simulink model "Multi_Scenario_WECS_based_Microgrid_2017"  (R2023a)
settings: Solver=ode45  StartTime=0.0  StopTime=4  RelTol=1e-3  EnableMultiTasking=on
undefined symbols (not defined in the file): c1, c2, c3, c4, c5, c6, DiscIntNeverNeededParam, fdesignblkfcn, gcbh, Hydride, Metal, Nickel
libraries: powerlib x63, powerlib_extras x26, powerlib_meascontrol x25, simulink x5, simulink_extras x2, electricdrivelib x1
(part 3 of 3)

== system Multi_Scenario_WECS_based_Microgrid_2017/Grid side control/Discrete PI Controller2 ==
  note: Discrete PID Controller
  note: Pierre Giroux, Gilbert Sybille
      | Power System Simulation Laboratory
      | IREQ, Hydro-Quebc
  Error : Inport  SampleTime=Ts
  Discrete-Time Integrator : DiscreteIntegrator  InitialCondition=Init  SampleTime=Ts  LimitOutput=on  UpperSaturationLimit=UpperLimit  LowerSaturationLimit=LowerLimit  ICPrevOutput=DiscIntNeverNeededParam  ICPrevScaledInput=DiscIntNeverNeededParam
  Kp4 : Gain  Gain=Kp  SaturateOnIntegerOverflow=on  SampleTime=Ts  OutDataTypeStr=Inherit: Same as input  ParamDataTypeStr=Inherit: Same as input
  Kp5 : Gain  Gain=Ki  SaturateOnIntegerOverflow=on  SampleTime=Ts  OutDataTypeStr=Inherit: Same as input  ParamDataTypeStr=Inherit: Same as input
  Saturation2 : Saturate  UpperLimit=UpperLimit  LowerLimit=LowerLimit  SampleTime=Ts
  Sum6 : Sum  InputSameDT=on  SaturateOnIntegerOverflow=on  SampleTime=Ts  OutDataTypeStr=Inherit: Same as first input
  Zero-Order Hold : ZeroOrderHold  SampleTime=Ts
  Out : Outport  SampleTime=Ts  InitialOutput=0
  wires:
  Zero-Order Hold/1 -> Sum6/1
  Saturation2/1 -> Out/1
  Discrete-Time Integrator/1 -> Sum6/2
  Kp4/1 -> Zero-Order Hold/1
  Kp5/1 -> Discrete-Time Integrator/1
  Sum6/1 -> Saturation2/1
  Error/1 -> Kp5/1, Kp4/1

== system Multi_Scenario_WECS_based_Microgrid_2017/Grid side control/Discrete PI Controller3 ==
  note: Pierre Giroux, Gilbert Sybille
      | Power System Simulation Laboratory
      | IREQ, Hydro-Quebc
  note: Discrete PID Controller
  Error : Inport  SampleTime=Ts
  Discrete-Time Integrator : DiscreteIntegrator  InitialCondition=Init  SampleTime=Ts  LimitOutput=on  UpperSaturationLimit=UpperLimit  LowerSaturationLimit=LowerLimit  ICPrevOutput=DiscIntNeverNeededParam  ICPrevScaledInput=DiscIntNeverNeededParam
  Kp4 : Gain  Gain=Kp  SaturateOnIntegerOverflow=on  SampleTime=Ts  OutDataTypeStr=Inherit: Same as input  ParamDataTypeStr=Inherit: Same as input
  Kp5 : Gain  Gain=Ki  SaturateOnIntegerOverflow=on  SampleTime=Ts  OutDataTypeStr=Inherit: Same as input  ParamDataTypeStr=Inherit: Same as input
  Saturation2 : Saturate  UpperLimit=UpperLimit  LowerLimit=LowerLimit  SampleTime=Ts
  Sum6 : Sum  InputSameDT=on  SaturateOnIntegerOverflow=on  SampleTime=Ts  OutDataTypeStr=Inherit: Same as first input
  Zero-Order Hold : ZeroOrderHold  SampleTime=Ts
  Out : Outport  SampleTime=Ts  InitialOutput=0
  wires:
  Error/1 -> Kp4/1, Kp5/1
  Sum6/1 -> Saturation2/1
  Kp5/1 -> Discrete-Time Integrator/1
  Kp4/1 -> Zero-Order Hold/1
  Discrete-Time Integrator/1 -> Sum6/2
  Saturation2/1 -> Out/1
  Zero-Order Hold/1 -> Sum6/1

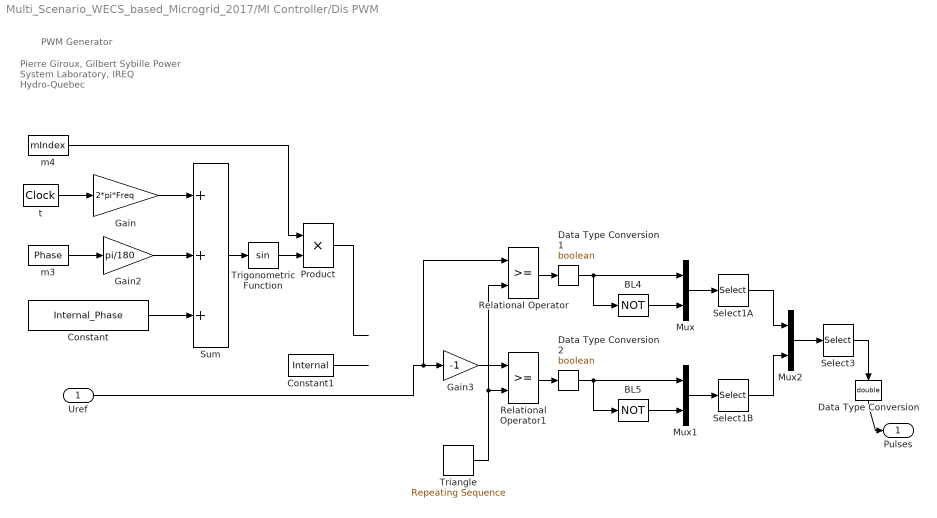
== system Multi_Scenario_WECS_based_Microgrid_2017/MI Controller/Dis PWM ==
  note: Pierre Giroux, Gilbert Sybille
      | Power System Laboratory, IREQ
      | Hydro-Quebec
  note: PWM Generator
  Uref : Inport
  BL4 : Logic  Operator=NOT  Inputs=1
  BL5 : Logic  Operator=NOT  Inputs=1
  Constant : Constant  Value=Internal_Phase
  Constant1 : Constant  Value=Internal
  Data Type Conversion : DataTypeConversion  OutDataTypeStr=double
  Data Type Conversion1 : DataTypeConversion  OutDataTypeStr=boolean
  Data Type Conversion2 : DataTypeConversion  OutDataTypeStr=boolean
  Gain : Gain  Gain=2*pi*Freq  SaturateOnIntegerOverflow=on  OutDataTypeStr=Inherit: Same as input  ParamDataTypeStr=Inherit: Same as input
  Gain2 : Gain  Gain=pi/180  SaturateOnIntegerOverflow=on  OutDataTypeStr=Inherit: Same as input  ParamDataTypeStr=Inherit: Same as input
  Gain3 : Gain  Gain=-1  SaturateOnIntegerOverflow=on  OutDataTypeStr=Inherit: Same as input  ParamDataTypeStr=Inherit: Same as input
  Mux : Mux  Inputs=2
  Mux1 : Mux  Inputs=2
  Mux2 : Mux  Inputs=2
  Product : Product  InputSameDT=on  SaturateOnIntegerOverflow=on  OutDataTypeStr=Inherit: Same as first input
  Relational Operator : RelationalOperator
  Relational Operator1 : RelationalOperator
  Select1A : Selector  InputPortWidth=Select1_PortWidth  IndexOptions=Index vector (dialog)  Indices=Select1_Elements  OutputSizes=1
  Select1B : Selector  InputPortWidth=Select1_PortWidth  IndexOptions=Index vector (dialog)  Indices=Select1_Elements  OutputSizes=1
  Select3 : Selector  InputPortWidth=Select3_PortWidth  IndexOptions=Index vector (dialog)  Indices=Select3_Elements  OutputSizes=1
  Sum : Sum  Inputs=+++  InputSameDT=on  SaturateOnIntegerOverflow=on  OutDataTypeStr=Inherit: Same as first input
  Triangle : simulink/Sources/Repeating Sequence  rep_seq_t=[0 1/Fc/4 3/Fc/4 1/Fc]  rep_seq_y=[0 -1 1 0]
  Trigonometric Function : Trigonometry
  m3 : Constant  Value=Phase
  m4 : Constant  Value=mIndex
  t : DigitalClock  SampleTime=Ts
  Pulses : Outport
  wires:
  Mux2/1 -> Select3/1
  Select1B/1 -> Mux2/2
  Select1A/1 -> Mux2/1
  Mux1/1 -> Select1B/1
  Mux/1 -> Select1A/1
  BL5/1 -> Mux1/2
  BL4/1 -> Mux/2
  Gain3/1 -> Relational Operator1/1
  Triangle/1 -> Relational Operator1/2, Relational Operator/2
  Product/1 -> ?
  Constant1/1 -> ?
  Uref/1 -> Relational Operator/1, Gain3/1
  Trigonometric Function/1 -> Product/2
  Sum/1 -> Trigonometric Function/1
  m4/1 -> Product/1
  Constant/1 -> Sum/3
  m3/1 -> Gain2/1
  Gain2/1 -> Sum/2
  Gain/1 -> Sum/1
  t/1 -> Gain/1
  Select3/1 -> Data Type Conversion/1
  Data Type Conversion/1 -> Pulses/1
  Relational Operator/1 -> Data Type Conversion1/1
  Data Type Conversion1/1 -> BL4/1, Mux/1
  Relational Operator1/1 -> Data Type Conversion2/1
  Data Type Conversion2/1 -> BL5/1, Mux1/1

== system Multi_Scenario_WECS_based_Microgrid_2017/MI Controller/Switch2 ==
  Vdq : Inport
  Compare To Constant1 : simulink/Logic and Bit Operations/Compare To Constant  relop=<  const=388  OutDataTypeStr=boolean
  Fcn1 : Fcn  Expr=sqrt(u(1)^2+u(2)^2)
  SW : Outport
  wires:
  Vdq/1 -> Fcn1/1
  Fcn1/1 -> Compare To Constant1/1
  Compare To Constant1/1 -> SW/1

== system Multi_Scenario_WECS_based_Microgrid_2017/MI Controller/central control ==
  Vdq_load : Inport
  Vdq_droop : Inport  Port=2
  Add1 : Sum
  Add2 : Sum
  Demux1 : Demux  Outputs=2
  Demux2 : Demux  Outputs=2
  Discrete PI Controller1 : powerlib_extras/Discrete  Control Blocks/Discrete PI Controller  Kp=0.2  Ki=40  Par_Limits=[100 -100]  Init=0  Ts=2e-05
  Discrete PI Controller2 : powerlib_extras/Discrete  Control Blocks/Discrete PI Controller  Kp=0.2  Ki=40  Par_Limits=[100 -100]  Init=0  Ts=2e-05
  Mux4 : Mux  Inputs=2
  Sum1 : Sum  Inputs=-+
  Sum2 : Sum  Inputs=-+
  v1 : Scope  NumInputPorts=2
  v5 : Scope  NumInputPorts=2
  out : Outport
  wires:
  Mux4/1 -> out/1
  Vdq_load/1 -> v1/1, Demux2/1
  Vdq_droop/1 -> v1/2, Demux1/1
  Demux2/1 -> Sum1/1
  Demux2/2 -> Sum2/1
  Sum1/1 -> Discrete PI Controller2/1
  Sum2/1 -> Discrete PI Controller1/1
  Demux1/2 -> Add2/2, Sum2/2
  Discrete PI Controller1/1 -> v5/2, Add2/1
  Discrete PI Controller2/1 -> v5/1, Add1/1
  Demux1/1 -> Add1/2, Sum1/2
  Add1/1 -> Mux4/1
  Add2/1 -> Mux4/2

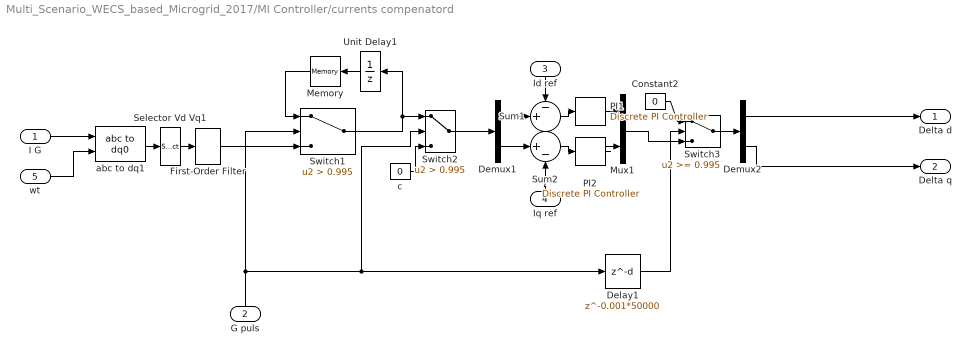
== system Multi_Scenario_WECS_based_Microgrid_2017/MI Controller/currents compenatord ==
  I G : Inport
  G puls : Inport  Port=2
  Id ref : Inport  Port=3
  Iq ref : Inport  Port=4
  wt : Inport  Port=5
  Constant2 : Constant  Value=0
  Delay1 : Delay  DelayLength=0.001*50000  InitialCondition=0  SampleTime=2e-05
  Demux1 : Demux  Outputs=2
  Demux2 : Demux  Outputs=2
  First-Order Filter : powerlib_meascontrol/Filters/First-Order Filter  FilterType=Lowpass  Tc=1e-3  Ts=0  Initialize=on  Vac_Init=[0, 0, 50]  Vdc_Init=0  PlotResponse=off  FreqRange="[0,  200,  1]"
  Memory : Memory
  Mux1 : Mux  Inputs=2
  "PI1 " : powerlib_extras/Discrete  Control Blocks/Discrete PI Controller  Kp=0.1  Ki=4  Par_Limits=[200 -200]  Init=0  Ts=2e-05
  PI2 : powerlib_extras/Discrete  Control Blocks/Discrete PI Controller  Kp=0.1  Ki=4  Par_Limits=[200 -200]  Init=0  Ts=2e-05
  Selector Vd Vq1 : Selector  InputPortWidth=3  IndexOptions=Index vector (dialog)  Indices=[1 2]  OutputSizes=1
  Sum1 : Sum  Inputs=-+|
  Sum2 : Sum  Inputs=|+-
  Switch1 : Switch  Criteria=u2 > Threshold  Threshold=0.995  SaturateOnIntegerOverflow=off  InputSameDT=off
  Switch2 : Switch  Criteria=u2 > Threshold  Threshold=0.995  SaturateOnIntegerOverflow=off  InputSameDT=off
  Switch3 : Switch  Threshold=0.995  SaturateOnIntegerOverflow=off  InputSameDT=off
  Unit Delay1 : UnitDelay  SampleTime=2e-05  HasFrameUpgradeWarning=on
  abc to dq1 : powerlib_meascontrol/Transformations/abc to dq0  Alignment=90 degrees behind phase A axis
  c : Constant  Value=0
  Delta d : Outport
  Delta q : Outport  Port=2
  wires:
  wt/1 -> abc to dq1/2
  Iq ref/1 -> Sum2/2
  Id ref/1 -> Sum1/1
  I G/1 -> abc to dq1/1
  abc to dq1/1 -> Selector Vd Vq1/1
  First-Order Filter/1 -> Switch1/3
  Switch1/1 -> Switch2/1, Unit Delay1/1
  Memory/1 -> Switch1/1
  Unit Delay1/1 -> Memory/1
  Demux1/1 -> Sum1/2
  Demux1/2 -> Sum2/1
  Sum2/1 -> PI2/1
  Sum1/1 -> "PI1 "/1
  Mux1/1 -> Switch3/3
  Demux2/1 -> Delta d/1
  Demux2/2 -> Delta q/1
  Switch3/1 -> Demux2/1
  Constant2/1 -> Switch3/1
  G puls/1 -> Switch2/2, Delay1/1, Switch1/2
  Selector Vd Vq1/1 -> First-Order Filter/1
  Delay1/1 -> Switch3/2
  "PI1 "/1 -> Mux1/1
  PI2/1 -> Mux1/2
  Switch2/1 -> Demux1/1
  c/1 -> Switch2/3

== system Multi_Scenario_WECS_based_Microgrid_2017/MI Controller/droop ==
  PQ : Inport
  Demux1 : Demux  Outputs=2
  Gain : Gain  Gain=2*pi
  Integrator : Integrator
  Pref : Constant  Value=180e3
  Subsystem1 : Subsystem
  Sum1 : Sum  Inputs=|+-
  Sum2 : Sum  Inputs=+-|
  Sum3 : Sum  Inputs=|-+
  Un : Constant  Value=390
  fn : Constant  Value=50
  m : Gain  Gain=6e-5
  n : Gain  Gain=4e-4
  Vabc : Outport
  wt : Outport  Port=2
  wires:
  Sum1/1 -> m/1
  fn/1 -> Sum2/1
  n/1 -> Sum2/2
  Sum2/1 -> Gain/1  "f"
  m/1 -> Sum3/1
  Un/1 -> Sum3/2
  Sum3/1 -> Subsystem1/2(Uref)
  Gain/1 -> Integrator/1  "w"
  Pref/1 -> Sum1/2
  Subsystem1/1(abc) -> Vabc/1
  Integrator/1 -> Subsystem1/1(wt), wt/1
  PQ/1 -> Demux1/1
  Demux1/1 -> Sum1/1
  Demux1/2 -> n/1

== system Multi_Scenario_WECS_based_Microgrid_2017/Wind Turbine model/cp(lambda,beta) ==
  lambda : Inport
  beta : Inport  Port=2
  Fcn : Fcn  Expr=1/(1/(u[1]+0.08*u[2])-0.035/(u[2]^3+1))
  Fcn1 : Fcn  Expr=c1*(c2/u[2]-c3*u[3]-c4)*exp(-c5/u[2])+c6*u[1]
  Mux : Mux  Inputs=2
  Mux1 : Mux  Inputs=3
  cp : Outport
  wires:
  Fcn/1 -> Mux1/2  "lambda_i"
  Fcn1/1 -> cp/1
  lambda/1 -> Mux1/1, Mux/1
  Mux1/1 -> Fcn1/1
  beta/1 -> Mux1/3, Mux/2
  Mux/1 -> Fcn/1

== system Multi_Scenario_WECS_based_Microgrid_2017/Wind-MPPT/Discrete PI Controller2 ==
  note: Pierre Giroux, Gilbert Sybille
      | Power System Simulation Laboratory
      | IREQ, Hydro-Quebc
  note: Discrete PID Controller
  Error : Inport  SampleTime=Ts
  Discrete-Time Integrator : DiscreteIntegrator  InitialCondition=Init  SampleTime=Ts  LimitOutput=on  UpperSaturationLimit=UpperLimit  LowerSaturationLimit=LowerLimit  ICPrevOutput=DiscIntNeverNeededParam  ICPrevScaledInput=DiscIntNeverNeededParam
  Kp4 : Gain  Gain=Kp  SaturateOnIntegerOverflow=on  SampleTime=Ts  OutDataTypeStr=Inherit: Same as input  ParamDataTypeStr=Inherit: Same as input
  Kp5 : Gain  Gain=Ki  SaturateOnIntegerOverflow=on  SampleTime=Ts  OutDataTypeStr=Inherit: Same as input  ParamDataTypeStr=Inherit: Same as input
  Saturation2 : Saturate  UpperLimit=UpperLimit  LowerLimit=LowerLimit  SampleTime=Ts
  Sum6 : Sum  InputSameDT=on  SaturateOnIntegerOverflow=on  SampleTime=Ts  OutDataTypeStr=Inherit: Same as first input
  Zero-Order Hold : ZeroOrderHold  SampleTime=Ts
  Out : Outport  SampleTime=Ts  InitialOutput=0
  wires:
  Error/1 -> Kp4/1, Kp5/1
  Sum6/1 -> Saturation2/1
  Kp5/1 -> Discrete-Time Integrator/1
  Kp4/1 -> Zero-Order Hold/1
  Discrete-Time Integrator/1 -> Sum6/2
  Saturation2/1 -> Out/1
  Zero-Order Hold/1 -> Sum6/1

== system Multi_Scenario_WECS_based_Microgrid_2017/Wind-MPPT/Pulse Generator ==
  Duty_Cycle : Inport
  Add : Sum  Inputs=-+
  Constant3 : Constant
  Constant4 : Constant  Value=0
  Digital Clock : DigitalClock  SampleTime=2e-05
  Divide2 : Product  Inputs=**
  Divide3 : Product  Inputs=**
  Math Function : Math  Operator=mod  SignedPower=on
  Nb_of_samples_by_cycle : Constant  Value=1/2000/2e-05
  Relational Operator1 : RelationalOperator  Operator=>  OutDataTypeStr=boolean  InputSameDT=off
  Rounding Function1 : Rounding  Operator=round
  Switch : Switch  Threshold=0.5  SaturateOnIntegerOverflow=off  InputSameDT=off
  Ts : Constant  Value=2e-05
  Pulse : Outport
  wires:
  Math Function/1 -> Relational Operator1/2
  Constant4/1 -> Switch/3
  Constant3/1 -> Switch/1
  Relational Operator1/1 -> Switch/2
  Nb_of_samples_by_cycle/1 -> Rounding Function1/1
  Divide2/1 -> Relational Operator1/1
  Divide3/1 -> Add/2, Math Function/2  "Period_of_cycle"
  Duty_Cycle/1 -> Divide2/1
  Rounding Function1/1 -> Divide3/2  "Nb_of_samples_by_cycle"
  Ts/1 -> Divide3/1, Add/1
  Digital Clock/1 -> Math Function/1
  Add/1 -> Divide2/2
  Switch/1 -> Pulse/1

== system Multi_Scenario_WECS_based_Microgrid_2017/Wind-MPPT/Torque reference 1 ==
  note: Inertia
  note: viscous damping
  wm : Inport
  1\ib1 : Gain  Gain=0.0024  SaturateOnIntegerOverflow=on  OutDataTypeStr=Inherit: Same as input  ParamDataTypeStr=Inherit: Same as input
  1\ib2 : Gain  Gain=0.4  SaturateOnIntegerOverflow=on  OutDataTypeStr=Inherit: Same as input  ParamDataTypeStr=Inherit: Same as input
  1\ib3 : Gain  Gain=0.01  SaturateOnIntegerOverflow=on  OutDataTypeStr=Inherit: Same as input  ParamDataTypeStr=Inherit: Same as input
  Add : Sum
  Differentiator Filter : Subsystem  DialogController=fdesignblkfcn  InitFcn=fdesignblkfcn(gcbh, {'InitFcn'});  mask(Differentiator Filter){}
      mask help: Design a differentiator filter
      settings: CopyFcn=fdesignblkfcn(gcbh, {'CopyFcn'});
      mask Help: helpview(mapfilelocation('dspblks'), 'dspdifferentiatorfilter')
      mask Display: disp('Differentiator');
  Math Function : Math  Operator=square  SignedPower=on
  Ref. sat.1 : Saturate  UpperLimit=inf  LowerLimit=0
  Subtract : Sum  Inputs=+-
  Tref : Outport
  wires:
  Math Function/1 -> 1\ib3/1
  wm/1 -> Math Function/1, Differentiator Filter/1(In), 1\ib1/1
  Ref. sat.1/1 -> Tref/1
  Differentiator Filter/1(Out) -> 1\ib2/1
  1\ib1/1 -> Add/2
  1\ib3/1 -> Subtract/1
  1\ib2/1 -> Add/1
  Subtract/1 -> Ref. sat.1/1
  Add/1 -> Subtract/2

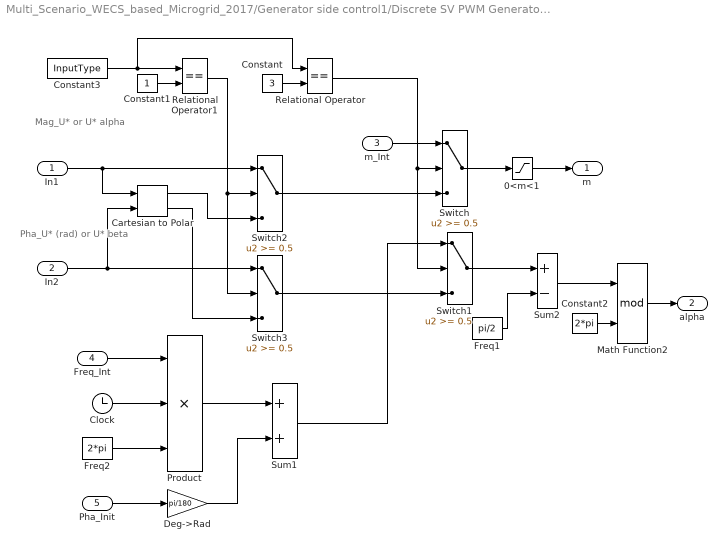
== system Multi_Scenario_WECS_based_Microgrid_2017/Generator side control1/Discrete SV PWM Generator/Determine reference vector (U*) ==
  note: Mag_U*
      | or
      | U* alpha
  note: Pha_U* (rad)
      | or
      | U* beta
  In1 : Inport
  In2 : Inport  Port=2
  m_Int : Inport  Port=3
  Freq_Int : Inport  Port=4
  Pha_Init : Inport  Port=5
  "0<m<1 " : Saturate  UpperLimit=1  LowerLimit=0
  Cartesian to Polar : simulink_extras/Transformations/Cartesian to Polar
  Clock : Clock
  Constant : Constant  Value=3
  Constant1 : Constant
  Constant2 : Constant  Value=2*pi
  Constant3 : Constant  Value=InputType
  Deg->Rad : Gain  Gain=pi/180  SaturateOnIntegerOverflow=on  OutDataTypeStr=Inherit: Same as input  ParamDataTypeStr=Inherit: Same as input
  Freq1 : Constant  Value=pi/2
  Freq2 : Constant  Value=2*pi
  Math Function2 : Math  Operator=mod  SignedPower=on
  Product : Product  Inputs=***  InputSameDT=on  SaturateOnIntegerOverflow=on  OutDataTypeStr=Inherit: Same as first input
  Relational Operator : RelationalOperator  Operator===  InputSameDT=off
  Relational Operator1 : RelationalOperator  Operator===  InputSameDT=off
  Sum1 : Sum  InputSameDT=on  SaturateOnIntegerOverflow=on  OutDataTypeStr=Inherit: Same as first input
  Sum2 : Sum  Inputs=+-  InputSameDT=on  SaturateOnIntegerOverflow=on  OutDataTypeStr=Inherit: Same as first input
  Switch{,1..3} (4 alike) : Switch  Threshold=0.5  InputSameDT=off
  m : Outport
  alpha : Outport  Port=2
  wires:
  Product/1 -> Sum1/1
  Pha_Init/1 -> Deg->Rad/1
  Deg->Rad/1 -> Sum1/2
  Freq_Int/1 -> Product/1
  Freq2/1 -> Product/3
  Switch/1 -> "0<m<1 "/1
  "0<m<1 "/1 -> m/1
  In1/1 -> Cartesian to Polar/1, Switch2/1
  In2/1 -> Cartesian to Polar/2, Switch3/1
  m_Int/1 -> Switch/1
  Constant/1 -> Relational Operator/2
  Relational Operator/1 -> Switch1/2, Switch/2
  Constant1/1 -> Relational Operator1/2
  Constant3/1 -> Relational Operator1/1, Relational Operator/1
  Switch2/1 -> Switch/3
  Cartesian to Polar/1 -> Switch2/3
  Cartesian to Polar/2 -> Switch3/3
  Switch3/1 -> Switch1/3
  Relational Operator1/1 -> Switch2/2, Switch3/2
  Clock/1 -> Product/2
  Constant2/1 -> Math Function2/2
  Math Function2/1 -> alpha/1
  Switch1/1 -> Sum2/1
  Sum1/1 -> Switch1/1
  Freq1/1 -> Sum2/2
  Sum2/1 -> Math Function2/1

== system Multi_Scenario_WECS_based_Microgrid_2017/Generator side control1/Discrete SV PWM Generator/INFO ==
  note: Two symmetrical switching patterns have been implemented:
  note: 3                       2
      |       3                   2
      |         3               2
      |           3           2
      |             3       2
      |               3   2
      | 4 4 4 4 4 4 4 4 0 1 1 1 1 1 1 1 1
      |               5   6
      |             5       6
      |           5           6
      |         5               6
      |       5                   6
      |     5                       6
  note: [1]
  note: [3]
  note: [4]
  note: [5]
  note: [6]
  note: U1 = 1 0 0
  note: U2 = 1 1 0
  note: U3 = 0 1 0
  note: U0 = 0 0 0
  note: U6 = 1 0 1
  note: U5 = 0 0 1
  note: U4 = 0 1 1
  note: Basic Space Vectors and Switching States
  note: [2]
  note: [n] = Sector number
  note: Vdc
  note: [Q1]
  note: [Q2]
  note: |
      | |
      | |
      | |
      | |
      | |
  note: |
      | |
      | |
  note: ---Va
  note: |
      | |
      | |
  note: [Q3]
  note: [Q4]
  note: |
      | |
      | |
      | |
      | |
      | |
  note: |
      | |
      | |
  note: ---Vb
  note: |
      | |
      | |
  note: [Q5]
  note: [Q6]
  note: |
      | |
      | |
      | |
      | |
      | |
  note: |
      | |
      | |
  note: ---Vc
  note: |
      | |
      | |
  note: --------------------------------------------------------
  note: +
  note: -
  note: Three-Phase VSC Diagram
  note: --------------------------------------------------------
  note: Q1 Q3 Q5
  note: U7 = 1 1 1
  note: The objective of the SV PWM technique is to approximate the reference voltage vector (U*) instantaneously
      | by combination of the switching states corresponding to the basic space vectors.
  note: Reference: Application Report SPRA524
      | Space-Vector PWM with TMS320C24x Using H/W & S/W Determined Switching Patterns
      | Zhenyu Yu, Texas Instruments
  note: --------------------------------------------------------------------------------------------------------------------------------------------------------------------
  note: Pattern #1:
      | With this pattern, identified as "Software-Determined" by Texas Instruments, each PWM channel switches twice per every PWM period.
  note: Pattern #2:
      | With this pattern, identified as "Hardware-Determined" by Texas Instruments, there is always one PWM channel staying constant for the entire PWM period.
      |  So the number of switching times for this pattern is less than pattern #1. As a result, switching losses will be reduced with Pattern #2.

== system Multi_Scenario_WECS_based_Microgrid_2017/Generator side control1/Discrete SV PWM Generator/SV Modulator Pattern #1 ==
  m : Inport
  alpha : Inport  Port=2
  Enable : EnablePort  PropagateVarSize=During execution
  "Compute time duration of switching states (Ta,Tb,To) " : Subsystem
  "Determine the sector of U* based on alpha (rad). Also, determine if the sector number is odd" : Subsystem
  Generate pulse pattern : Subsystem
      mask init:
      | %Switching pattern:
      | pat1=[0 1 1 1 1 1 0;0 0 1 1 1 0 0;0 0 0 1 0 0 0];
      | pat1(:,:,2)=[0 0 1 1 1 0 0;0 1 1 1 1 1 0;0 0 0 1 0 0 0];
      | pat1(:,:,3)=[0 0 0 1 0 0 0;0 1 1 1 1 1 0;0 0 1 1 1 0 0];
      | pat1(:,:,4)=[0 0 0 1 0 0 0;0 0 1 1 1 0 0;0 1 1 1 1 1 0];
      | pat1(:,:,5)=[0 0 1 1 1 0 0;0 0 0 1 0 0 0;0 1 1 1 1 1 0];
      | pat1(:,:,6)=[0 1 1 1 1 1 0;0 0 0 1 0 0 0;0 0 1 1 1 0 0];
  INFO : Subsystem
      mask Display: disp('?')
  Pulses : Outport
  wires:
  "Determine the sector of U* based on alpha (rad). Also, determine if the sector number is odd"/1(Sn) -> "Compute time duration of switching states (Ta,Tb,To) "/3(Sn), Generate pulse pattern/1(Sn)
  "Determine the sector of U* based on alpha (rad). Also, determine if the sector number is odd"/2(Odd_S) -> "Compute time duration of switching states (Ta,Tb,To) "/4(Odd_S)
  "Compute time duration of switching states (Ta,Tb,To) "/1(Ta_Tb_To) -> Generate pulse pattern/2(TaTbTo)
  Generate pulse pattern/1(Pulses) -> Pulses/1
  alpha/1 -> "Determine the sector of U* based on alpha (rad). Also, determine if the sector number is odd"/1(alpha), "Compute time duration of switching states (Ta,Tb,To) "/1(alpha)
  m/1 -> "Compute time duration of switching states (Ta,Tb,To) "/2(m)

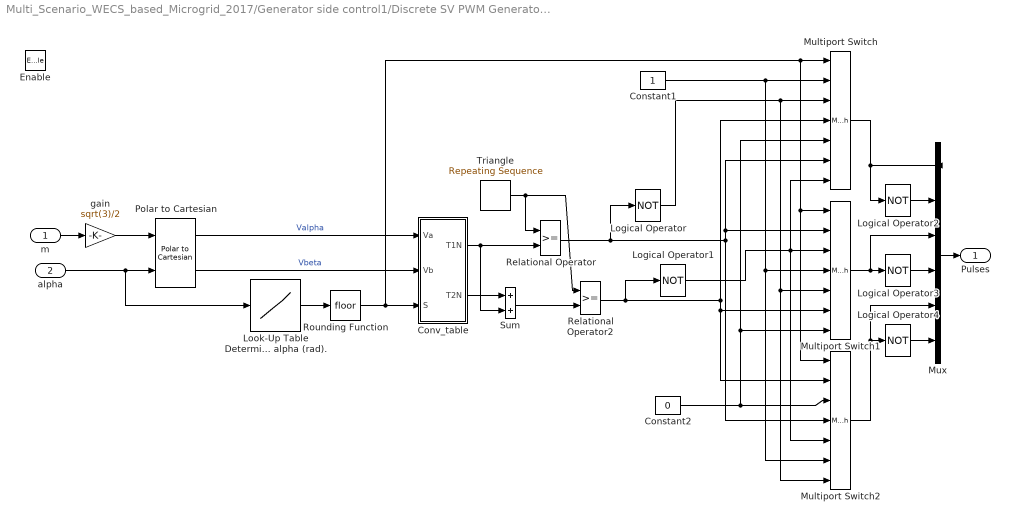
== system Multi_Scenario_WECS_based_Microgrid_2017/Generator side control1/Discrete SV PWM Generator/SV Modulator Pattern #2 ==
  m : Inport
  alpha : Inport  Port=2
  Enable : EnablePort  PropagateVarSize=During execution
  Constant1 : Constant
  Constant2 : Constant  Value=0
  Conv_table : Subsystem
  Logical Operator{,1..4} (5 alike) : Logic  Operator=NOT  OutDataTypeStr=float('double')
  "Look-Up Table Determine the sector of U* based on alpha (rad). " : Lookup  InputValues=[0:pi/3:5*pi/3]  Table=[1:6]
  Multiport Switch : MultiPortSwitch  Inputs=6
  Multiport Switch1 : MultiPortSwitch  Inputs=6
  Multiport Switch2 : MultiPortSwitch  Inputs=6
  Mux : Mux  Inputs=6
  Polar to Cartesian : simulink_extras/Transformations/Polar to Cartesian
  Relational Operator : RelationalOperator  OutDataTypeStr=float('double')
  Relational Operator2 : RelationalOperator  OutDataTypeStr=float('double')
  Rounding Function : Rounding
  Sum : Sum  InputSameDT=on  SaturateOnIntegerOverflow=on  OutDataTypeStr=Inherit: Same as first input
  Triangle : simulink/Sources/Repeating Sequence  rep_seq_t=[0 0.5/Fc 1/Fc]  rep_seq_y=[0 1 0]
  gain : Gain  Gain=sqrt(3)/2  SaturateOnIntegerOverflow=on  OutDataTypeStr=Inherit: Same as input  ParamDataTypeStr=Inherit: Same as input
  Pulses : Outport
  wires:
  gain/1 -> Polar to Cartesian/1
  alpha/1 -> Polar to Cartesian/2, "Look-Up Table Determine the sector of U* based on alpha (rad). "/1
  m/1 -> gain/1
  Polar to Cartesian/2 -> Conv_table/2(Vb)  "Vbeta"
  Polar to Cartesian/1 -> Conv_table/1(Va)  "Valpha"
  Constant2/1 -> Multiport Switch1/7, Multiport Switch/5, Multiport Switch2/3
  Logical Operator1/1 -> Multiport Switch/7, Multiport Switch2/5, Multiport Switch1/3
  Logical Operator/1 -> Multiport Switch2/7, Multiport Switch1/5, Multiport Switch/3
  Relational Operator2/1 -> Multiport Switch1/6, Multiport Switch2/2, Multiport Switch/4, Logical Operator1/1
  Relational Operator/1 -> Multiport Switch/6, Multiport Switch1/2, Multiport Switch2/4, Logical Operator/1
  Constant1/1 -> Multiport Switch2/6, Multiport Switch1/4, Multiport Switch/2
  Triangle/1 -> Relational Operator/1, Relational Operator2/1
  Sum/1 -> Relational Operator2/2
  Conv_table/2(T2N) -> Sum/1
  Conv_table/1(T1N) -> Sum/2, Relational Operator/2
  Logical Operator2/1 -> Mux/2
  Logical Operator3/1 -> Mux/4
  Logical Operator4/1 -> Mux/6
  Multiport Switch/1 -> Mux/1, Logical Operator2/1
  Multiport Switch1/1 -> Mux/3, Logical Operator3/1
  Multiport Switch2/1 -> Mux/5, Logical Operator4/1
  Mux/1 -> Pulses/1
  Rounding Function/1 -> Multiport Switch2/1, Multiport Switch1/1, Multiport Switch/1, Conv_table/3(S)
  "Look-Up Table Determine the sector of U* based on alpha (rad). "/1 -> Rounding Function/1

== system Multi_Scenario_WECS_based_Microgrid_2017/MI Controller/droop/Subsystem1 ==
  wt : Inport
  Uref : Inport  Port=2
  Add : Sum  Inputs=+-
  Add1 : Sum
  Constant : Constant  Value=2*pi/3
  Mux : Mux  Inputs=3
  Product : Product  RndMeth=Zero
  Product1 : Product  RndMeth=Zero
  Product2 : Product  RndMeth=Zero
  Trigonometric Function : Trigonometry
  Trigonometric Function1 : Trigonometry
  Trigonometric Function2 : Trigonometry
  abc : Outport
  wires:
  Constant/1 -> Add1/2, Add/2
  Trigonometric Function2/1 -> Product2/2
  Add/1 -> Trigonometric Function1/1
  Product1/1 -> Mux/2
  wt/1 -> Trigonometric Function/1, Add1/1, Add/1
  Add1/1 -> Trigonometric Function2/1
  Trigonometric Function/1 -> Product/2
  Uref/1 -> Product2/1, Product1/1, Product/1
  Trigonometric Function1/1 -> Product1/2
  Mux/1 -> abc/1
  Product2/1 -> Mux/3
  Product/1 -> Mux/1

== system Multi_Scenario_WECS_based_Microgrid_2017/Wind-MPPT/Torque reference 1/Differentiator Filter ==
  In : Inport
  Generated Filter Block : Subsystem  Tag=FilterWizardSubSystem
      settings: ErrorFcn=dspFilterRealizedInBasicElemsAlgLoopErrFcnCallback
  Out : Outport
  wires:
  Generated Filter Block/1(Output) -> Out/1
  In/1 -> Generated Filter Block/1(Input)

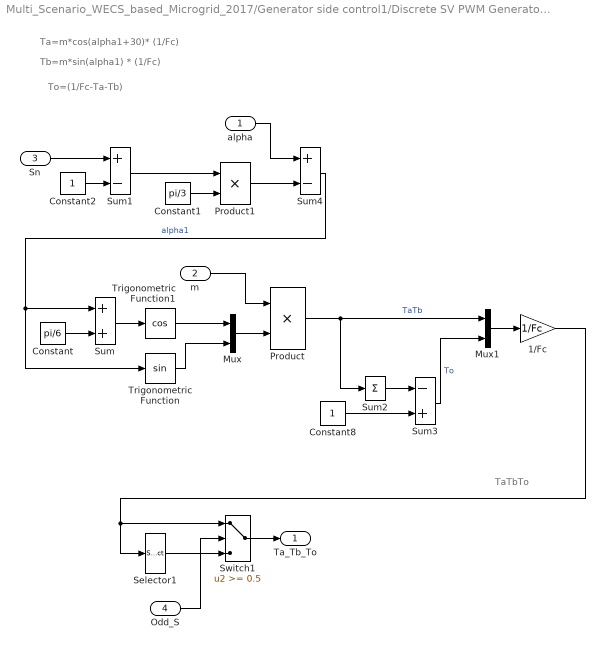
== system Multi_Scenario_WECS_based_Microgrid_2017/Generator side control1/Discrete SV PWM Generator/SV Modulator Pattern #1/Compute time duration of switching states (Ta,Tb,To)  ==
  note: Ta=m*cos(alpha1+30)* (1/Fc)
  note: Tb=m*sin(alpha1) * (1/Fc)
  note: To=(1/Fc-Ta-Tb)
  note: TaTbTo
  alpha : Inport
  m : Inport  Port=2
  Sn : Inport  Port=3
  Odd_S : Inport  Port=4
  1/Fc : Gain  Gain=1/Fc  SaturateOnIntegerOverflow=on  OutDataTypeStr=Inherit: Same as input  ParamDataTypeStr=Inherit: Same as input
  Constant : Constant  Value=pi/6
  Constant1 : Constant  Value=pi/3
  Constant2 : Constant
  Constant8 : Constant
  Mux : Mux  Inputs=2
  Mux1 : Mux  Inputs=2
  Product : Product  SaturateOnIntegerOverflow=on  OutDataTypeStr=Inherit: Same as first input
  Product1 : Product  SaturateOnIntegerOverflow=on  OutDataTypeStr=Inherit: Same as first input
  Selector1 : Selector  InputPortWidth=3  IndexOptions=Index vector (dialog)  Indices=[2 1 3]  OutputSizes=1
  Sum : Sum  SaturateOnIntegerOverflow=on
  Sum1 : Sum  Inputs=+-  SaturateOnIntegerOverflow=on
  Sum2 : Sum  Inputs=1  SaturateOnIntegerOverflow=on
  Sum3 : Sum  Inputs=-+  SaturateOnIntegerOverflow=on
  Sum4 : Sum  Inputs=+-  SaturateOnIntegerOverflow=on
  Switch1 : Switch  Threshold=0.5  InputSameDT=off
  Trigonometric Function : Trigonometry
  Trigonometric Function1 : Trigonometry  Operator=cos
  Ta_Tb_To : Outport
  wires:
  Trigonometric Function1/1 -> Mux/1
  Trigonometric Function/1 -> Mux/2
  Mux/1 -> Product/2
  m/1 -> Product/1
  Sum/1 -> Trigonometric Function1/1
  Sum2/1 -> Sum3/1
  Constant8/1 -> Sum3/2
  Sum1/1 -> Product1/1
  Constant1/1 -> Product1/2
  Sn/1 -> Sum1/1
  Constant2/1 -> Sum1/2
  Product1/1 -> Sum4/2
  alpha/1 -> Sum4/1
  Product/1 -> Mux1/1, Sum2/1  "TaTb"
  Sum3/1 -> Mux1/2  "To"
  Mux1/1 -> 1/Fc/1
  Sum4/1 -> Sum/1, Trigonometric Function/1  "alpha1"
  Constant/1 -> Sum/2
  1/Fc/1 -> Switch1/1, Selector1/1
  Selector1/1 -> Switch1/3
  Switch1/1 -> Ta_Tb_To/1
  Odd_S/1 -> Switch1/2

== system Multi_Scenario_WECS_based_Microgrid_2017/Generator side control1/Discrete SV PWM Generator/SV Modulator Pattern #1/Determine the sector of U* based on alpha (rad). Also, determine if the sector number is odd ==
  alpha : Inport
  Constant1 : Constant  Value=2
  Look-Up Table : Lookup  InputValues=[0:pi/3:5*pi/3]  Table=[1:6]
  Math Function1 : Math  Operator=mod  SignedPower=on
  Rounding Function : Rounding
  Sn : Outport
  Odd_S : Outport  Port=2
  wires:
  Look-Up Table/1 -> Rounding Function/1
  Rounding Function/1 -> Math Function1/1, Sn/1
  Constant1/1 -> Math Function1/2
  Math Function1/1 -> Odd_S/1
  alpha/1 -> Look-Up Table/1

== system Multi_Scenario_WECS_based_Microgrid_2017/Generator side control1/Discrete SV PWM Generator/SV Modulator Pattern #1/Generate pulse pattern ==
  note: Page-> based on which time interval (1 to 7) of the PWM period
  note: Column-> pulses for Q1,Q3 et Q5 based on Sector number
  Sn : Inport
  TaTbTo : Inport  Port=2
  Constant2 : Constant
  Constant3 : Constant
  Determine interval of the PWM period based on Ta Tb and To : Subsystem
  Direct Look-Up Table (n-D) : LookupNDDirect  NumberOfTableDimensions=3  InputsSelectThisObjectFromTable=Vector  Table=pat1
  Logical Operator : Logic  Operator=NOT  AllPortsSameDT=off  OutDataTypeStr=float('double')
  Mux : Mux  Inputs=[3 3]
  Selector : Selector  InputPortWidth=6  IndexOptions=Index vector (dialog)  Indices=[1 4 2 5 3 6]  OutputSizes=1
  Sum : Sum  Inputs=+-  SaturateOnIntegerOverflow=on
  Sum1 : Sum  Inputs=+-  SaturateOnIntegerOverflow=on
  Pulses : Outport
  wires:
  Determine interval of the PWM period based on Ta Tb and To/1(Tn) -> Sum/1  "Interval n"
  Selector/1 -> Pulses/1
  Mux/1 -> Selector/1
  Logical Operator/1 -> Mux/2  "Q2 Q4 Q6"
  Direct Look-Up Table (n-D)/1 -> Logical Operator/1, Mux/1  "Q1 Q3 Q5"
  Sum1/1 -> Direct Look-Up Table (n-D)/2  "Column"
  Sn/1 -> Sum1/1
  Constant3/1 -> Sum1/2
  Sum/1 -> Direct Look-Up Table (n-D)/1  "Page"
  Constant2/1 -> Sum/2
  TaTbTo/1 -> Determine interval of the PWM period based on Ta Tb and To/1(TaTbTo)

== system Multi_Scenario_WECS_based_Microgrid_2017/Generator side control1/Discrete SV PWM Generator/SV Modulator Pattern #1/INFO ==
  note: where:
      | Fc = Chopping frequency
      | m = modulation index
      | alpha = angle between reference vector U* and
      | 1st basic space vector
  note: To=(1/Fc-Ta-Tb)
  note: Tb=m*sin(alpha) * (1/Fc)
  note: Ta=m*cos(alpha+30)* (1/Fc)
  note: To/4
  note: Ta/2
  note: Tb/2
  note: To/2
  note: Tb/2
  note: To/4
  note: Ta/2
  note: |
      | |
      | |
      | |
      | |
      | |
      | |
      | |
      | |
      | |
  note: |
      | |
      | |
      | |
      | |
      | |
      | |
      | |
      | |
      | |
  note: |
      | |
      | |
      | |
      | |
      | |
      | |
      | |
      | |
      | |
  note: |
      | |
      | |
      | |
      | |
      | |
      | |
      | |
      | |
      | |
  note: |
      | |
      | |
      | |
      | |
      | |
      | |
      | |
      | |
      | |
  note: |
      | |
      | |
      | |
      | |
      | |
      | |
      | |
      | |
      | |
  note: Pattern #1 implements the following symmetrical switching pattern:
      | total duration = 1 PWM period (Tpwm = 1/Fc)
  note: 1st basic
      | space vector
  note: 2nd basic
      | space vector
  note: zero
      | space vector
      | (Q1 Q3 Q5 =0)
  note: zero
      | space vector
      | (Q1 Q3 Q5 =1)
  note: 2nd basic
      | space vector
  note: 1st basic
      | space vector
  note: zero
      | space vector
      | (Q1 Q3 Q5 =0)
  note: Interval 1
  note: Interval 2
  note: Interval 3
  note: Interval 4
  note: Interval 5
  note: Interval 6
  note: Interval 7

== system Multi_Scenario_WECS_based_Microgrid_2017/Generator side control1/Discrete SV PWM Generator/SV Modulator Pattern #2/Conv_table ==
  Va : Inport
  Vb : Inport  Port=2
  S : Inport  Port=3
  Look-Up Table : Lookup  InputValues=[1 2 3 4 5 6]  Table=[1 1 0 -1 -1 0]
  Look-Up Table1 : Lookup  InputValues=[1 2 3 4 5 6]  Table=[-1/sqrt(3) 1/sqrt(3) 2/sqrt(3) 1/sqrt(3) -1/sqrt(3) -2/sqrt(3)]
  Look-Up Table2 : Lookup  InputValues=[1 2 3 4 5 6]  Table=[0 -1 -1 0 1 1]
  Look-Up Table3 : Lookup  InputValues=[1 2 3 4 5 6]  Table=[2/sqrt(3) 1/sqrt(3) -1/sqrt(3) -2/sqrt(3) -1/sqrt(3) 1/sqrt(3)]
  Product{,1..3} (4 alike) : Product  InputSameDT=on  SaturateOnIntegerOverflow=on  OutDataTypeStr=Inherit: Same as first input
  Sum : Sum  InputSameDT=on  SaturateOnIntegerOverflow=on  OutDataTypeStr=Inherit: Same as first input
  Sum1 : Sum  InputSameDT=on  SaturateOnIntegerOverflow=on  OutDataTypeStr=Inherit: Same as first input
  T1N : Outport
  T2N : Outport  Port=2
  wires:
  Sum1/1 -> T2N/1
  Sum/1 -> T1N/1
  Product3/1 -> Sum1/2
  Product2/1 -> Sum1/1
  Product1/1 -> Sum/2
  Product/1 -> Sum/1
  Look-Up Table3/1 -> Product3/2
  Look-Up Table2/1 -> Product2/2
  Look-Up Table1/1 -> Product1/2
  Vb/1 -> Product3/1, Product1/1
  Look-Up Table/1 -> Product/2
  Va/1 -> Product2/1, Product/1
  S/1 -> Look-Up Table1/1, Look-Up Table2/1, Look-Up Table3/1, Look-Up Table/1

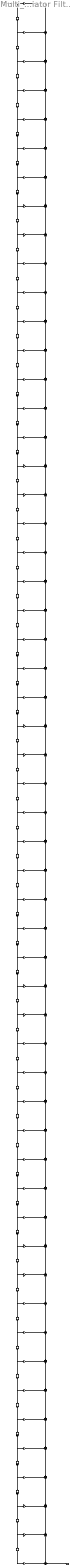
== system Multi_Scenario_WECS_based_Microgrid_2017/Wind-MPPT/Torque reference 1/Differentiator Filter/Generated Filter Block ==
  Input : Inport
  BodyDelay{2..55} (54 alike) : Delay  DelayLength=1  InitialCondition=0
  BodyLSum{2..55} (54 alike) : Sum  Inputs=++|  RndMeth=Nearest  SaturateOnIntegerOverflow=on  OutDataTypeStr=Inherit: Same as first input
  b(1) : Gain  Gain=0.0016485839041717814  ParamDataTypeStr=double  RndMeth=Nearest  SaturateOnIntegerOverflow=on  OutDataTypeStr=Inherit: Same as input
  b(10) : Gain  Gain=0.011014879869749038  ParamDataTypeStr=double  RndMeth=Nearest  SaturateOnIntegerOverflow=on  OutDataTypeStr=Inherit: Same as input
  b(11) : Gain  Gain=-0.005763535930488289  ParamDataTypeStr=double  RndMeth=Nearest  SaturateOnIntegerOverflow=on  OutDataTypeStr=Inherit: Same as input
  b(12) : Gain  Gain=-0.015198183055521291  ParamDataTypeStr=double  RndMeth=Nearest  SaturateOnIntegerOverflow=on  OutDataTypeStr=Inherit: Same as input
  b(13) : Gain  Gain=0.0065686388642668125  ParamDataTypeStr=double  RndMeth=Nearest  SaturateOnIntegerOverflow=on  OutDataTypeStr=Inherit: Same as input
  b(14) : Gain  Gain=0.020867949959447685  ParamDataTypeStr=double  RndMeth=Nearest  SaturateOnIntegerOverflow=on  OutDataTypeStr=Inherit: Same as input
  b(15) : Gain  Gain=-0.0070602627960907761  ParamDataTypeStr=double  RndMeth=Nearest  SaturateOnIntegerOverflow=on  OutDataTypeStr=Inherit: Same as input
  b(16) : Gain  Gain=-0.028242635943863115  ParamDataTypeStr=double  RndMeth=Nearest  SaturateOnIntegerOverflow=on  OutDataTypeStr=Inherit: Same as input
  b(17) : Gain  Gain=0.0072704924773104602  ParamDataTypeStr=double  RndMeth=Nearest  SaturateOnIntegerOverflow=on  OutDataTypeStr=Inherit: Same as input
  b(18) : Gain  Gain=0.038329320446368831  ParamDataTypeStr=double  RndMeth=Nearest  SaturateOnIntegerOverflow=on  OutDataTypeStr=Inherit: Same as input
  b(19) : Gain  Gain=-0.0068002265270407335  ParamDataTypeStr=double  RndMeth=Nearest  SaturateOnIntegerOverflow=on  OutDataTypeStr=Inherit: Same as input
  b(2) : Gain  Gain=0.00017042943589109515  ParamDataTypeStr=double  RndMeth=Nearest  SaturateOnIntegerOverflow=on  OutDataTypeStr=Inherit: Same as input
  b(20) : Gain  Gain=-0.052819993002155979  ParamDataTypeStr=double  RndMeth=Nearest  SaturateOnIntegerOverflow=on  OutDataTypeStr=Inherit: Same as input
  b(21) : Gain  Gain=0.0049482783503700303  ParamDataTypeStr=double  RndMeth=Nearest  SaturateOnIntegerOverflow=on  OutDataTypeStr=Inherit: Same as input
  b(22) : Gain  Gain=0.075871674298216854  ParamDataTypeStr=double  RndMeth=Nearest  SaturateOnIntegerOverflow=on  OutDataTypeStr=Inherit: Same as input
  b(23) : Gain  Gain=0.00073312852370663187  ParamDataTypeStr=double  RndMeth=Nearest  SaturateOnIntegerOverflow=on  OutDataTypeStr=Inherit: Same as input
  b(24) : Gain  Gain=-0.11992357305817197  ParamDataTypeStr=double  RndMeth=Nearest  SaturateOnIntegerOverflow=on  OutDataTypeStr=Inherit: Same as input
  b(25) : Gain  Gain=-0.022982436984387573  ParamDataTypeStr=double  RndMeth=Nearest  SaturateOnIntegerOverflow=on  OutDataTypeStr=Inherit: Same as input
  b(26) : Gain  Gain=0.24743192698089661  ParamDataTypeStr=double  RndMeth=Nearest  SaturateOnIntegerOverflow=on  OutDataTypeStr=Inherit: Same as input
  b(27) : Gain  Gain=0.30572927022108959  ParamDataTypeStr=double  RndMeth=Nearest  SaturateOnIntegerOverflow=on  OutDataTypeStr=Inherit: Same as input
  b(28) : Gain  Gain=0  ParamDataTypeStr=double  RndMeth=Nearest  SaturateOnIntegerOverflow=on  OutDataTypeStr=Inherit: Same as input
  b(29) : Gain  Gain=-0.30572927022108959  ParamDataTypeStr=double  RndMeth=Nearest  SaturateOnIntegerOverflow=on  OutDataTypeStr=Inherit: Same as input
  b(3) : Gain  Gain=-0.0038948238157296474  ParamDataTypeStr=double  RndMeth=Nearest  SaturateOnIntegerOverflow=on  OutDataTypeStr=Inherit: Same as input
  b(30) : Gain  Gain=-0.24743192698089661  ParamDataTypeStr=double  RndMeth=Nearest  SaturateOnIntegerOverflow=on  OutDataTypeStr=Inherit: Same as input
  b(31) : Gain  Gain=0.022982436984387573  ParamDataTypeStr=double  RndMeth=Nearest  SaturateOnIntegerOverflow=on  OutDataTypeStr=Inherit: Same as input
  b(32) : Gain  Gain=0.11992357305817197  ParamDataTypeStr=double  RndMeth=Nearest  SaturateOnIntegerOverflow=on  OutDataTypeStr=Inherit: Same as input
  b(33) : Gain  Gain=-0.00073312852370663187  ParamDataTypeStr=double  RndMeth=Nearest  SaturateOnIntegerOverflow=on  OutDataTypeStr=Inherit: Same as input
  b(34) : Gain  Gain=-0.075871674298216854  ParamDataTypeStr=double  RndMeth=Nearest  SaturateOnIntegerOverflow=on  OutDataTypeStr=Inherit: Same as input
  b(35) : Gain  Gain=-0.0049482783503700303  ParamDataTypeStr=double  RndMeth=Nearest  SaturateOnIntegerOverflow=on  OutDataTypeStr=Inherit: Same as input
  b(36) : Gain  Gain=0.052819993002155979  ParamDataTypeStr=double  RndMeth=Nearest  SaturateOnIntegerOverflow=on  OutDataTypeStr=Inherit: Same as input
  b(37) : Gain  Gain=0.0068002265270407335  ParamDataTypeStr=double  RndMeth=Nearest  SaturateOnIntegerOverflow=on  OutDataTypeStr=Inherit: Same as input
  b(38) : Gain  Gain=-0.038329320446368831  ParamDataTypeStr=double  RndMeth=Nearest  SaturateOnIntegerOverflow=on  OutDataTypeStr=Inherit: Same as input
  b(39) : Gain  Gain=-0.0072704924773104602  ParamDataTypeStr=double  RndMeth=Nearest  SaturateOnIntegerOverflow=on  OutDataTypeStr=Inherit: Same as input
  b(4) : Gain  Gain=-0.0032830177673830903  ParamDataTypeStr=double  RndMeth=Nearest  SaturateOnIntegerOverflow=on  OutDataTypeStr=Inherit: Same as input
  b(40) : Gain  Gain=0.028242635943863115  ParamDataTypeStr=double  RndMeth=Nearest  SaturateOnIntegerOverflow=on  OutDataTypeStr=Inherit: Same as input
  b(41) : Gain  Gain=0.0070602627960907761  ParamDataTypeStr=double  RndMeth=Nearest  SaturateOnIntegerOverflow=on  OutDataTypeStr=Inherit: Same as input
  b(42) : Gain  Gain=-0.020867949959447685  ParamDataTypeStr=double  RndMeth=Nearest  SaturateOnIntegerOverflow=on  OutDataTypeStr=Inherit: Same as input
  b(43) : Gain  Gain=-0.0065686388642668125  ParamDataTypeStr=double  RndMeth=Nearest  SaturateOnIntegerOverflow=on  OutDataTypeStr=Inherit: Same as input
  b(44) : Gain  Gain=0.015198183055521291  ParamDataTypeStr=double  RndMeth=Nearest  SaturateOnIntegerOverflow=on  OutDataTypeStr=Inherit: Same as input
  b(45) : Gain  Gain=0.005763535930488289  ParamDataTypeStr=double  RndMeth=Nearest  SaturateOnIntegerOverflow=on  OutDataTypeStr=Inherit: Same as input
  b(46) : Gain  Gain=-0.011014879869749038  ParamDataTypeStr=double  RndMeth=Nearest  SaturateOnIntegerOverflow=on  OutDataTypeStr=Inherit: Same as input
  b(47) : Gain  Gain=-0.0051172092513206112  ParamDataTypeStr=double  RndMeth=Nearest  SaturateOnIntegerOverflow=on  OutDataTypeStr=Inherit: Same as input
  b(48) : Gain  Gain=0.0075034408734532933  ParamDataTypeStr=double  RndMeth=Nearest  SaturateOnIntegerOverflow=on  OutDataTypeStr=Inherit: Same as input
  b(49) : Gain  Gain=0.0039498824016694347  ParamDataTypeStr=double  RndMeth=Nearest  SaturateOnIntegerOverflow=on  OutDataTypeStr=Inherit: Same as input
  b(5) : Gain  Gain=0.0039854203993547783  ParamDataTypeStr=double  RndMeth=Nearest  SaturateOnIntegerOverflow=on  OutDataTypeStr=Inherit: Same as input
  b(50) : Gain  Gain=-0.0056185919166623251  ParamDataTypeStr=double  RndMeth=Nearest  SaturateOnIntegerOverflow=on  OutDataTypeStr=Inherit: Same as input
  b(51) : Gain  Gain=-0.0039854203993547783  ParamDataTypeStr=double  RndMeth=Nearest  SaturateOnIntegerOverflow=on  OutDataTypeStr=Inherit: Same as input
  b(52) : Gain  Gain=0.0032830177673830903  ParamDataTypeStr=double  RndMeth=Nearest  SaturateOnIntegerOverflow=on  OutDataTypeStr=Inherit: Same as input
  b(53) : Gain  Gain=0.0038948238157296474  ParamDataTypeStr=double  RndMeth=Nearest  SaturateOnIntegerOverflow=on  OutDataTypeStr=Inherit: Same as input
  b(54) : Gain  Gain=-0.00017042943589109515  ParamDataTypeStr=double  RndMeth=Nearest  SaturateOnIntegerOverflow=on  OutDataTypeStr=Inherit: Same as input
  b(55) : Gain  Gain=-0.0016485839041717814  ParamDataTypeStr=double  RndMeth=Nearest  SaturateOnIntegerOverflow=on  OutDataTypeStr=Inherit: Same as input
  b(6) : Gain  Gain=0.0056185919166623251  ParamDataTypeStr=double  RndMeth=Nearest  SaturateOnIntegerOverflow=on  OutDataTypeStr=Inherit: Same as input
  b(7) : Gain  Gain=-0.0039498824016694347  ParamDataTypeStr=double  RndMeth=Nearest  SaturateOnIntegerOverflow=on  OutDataTypeStr=Inherit: Same as input
  b(8) : Gain  Gain=-0.0075034408734532933  ParamDataTypeStr=double  RndMeth=Nearest  SaturateOnIntegerOverflow=on  OutDataTypeStr=Inherit: Same as input
  b(9) : Gain  Gain=0.0051172092513206112  ParamDataTypeStr=double  RndMeth=Nearest  SaturateOnIntegerOverflow=on  OutDataTypeStr=Inherit: Same as input
  Output : Outport
  wires:
  Input/1 -> b(1)/1, BodyDelay2/1
  b(1)/1 -> BodyLSum2/2
  BodyDelay2/1 -> b(2)/1, BodyDelay3/1
  b(2)/1 -> BodyLSum2/1
  BodyLSum2/1 -> BodyLSum3/2
  BodyDelay3/1 -> b(3)/1, BodyDelay4/1
  b(3)/1 -> BodyLSum3/1
  BodyLSum3/1 -> BodyLSum4/2
  BodyDelay4/1 -> b(4)/1, BodyDelay5/1
  b(4)/1 -> BodyLSum4/1
  BodyLSum4/1 -> BodyLSum5/2
  BodyDelay5/1 -> b(5)/1, BodyDelay6/1
  b(5)/1 -> BodyLSum5/1
  BodyLSum5/1 -> BodyLSum6/2
  BodyDelay6/1 -> b(6)/1, BodyDelay7/1
  b(6)/1 -> BodyLSum6/1
  BodyLSum6/1 -> BodyLSum7/2
  BodyDelay7/1 -> b(7)/1, BodyDelay8/1
  b(7)/1 -> BodyLSum7/1
  BodyLSum7/1 -> BodyLSum8/2
  BodyDelay8/1 -> b(8)/1, BodyDelay9/1
  b(8)/1 -> BodyLSum8/1
  BodyLSum8/1 -> BodyLSum9/2
  BodyDelay9/1 -> b(9)/1, BodyDelay10/1
  b(9)/1 -> BodyLSum9/1
  BodyLSum9/1 -> BodyLSum10/2
  BodyDelay10/1 -> b(10)/1, BodyDelay11/1
  b(10)/1 -> BodyLSum10/1
  BodyLSum10/1 -> BodyLSum11/2
  BodyDelay11/1 -> b(11)/1, BodyDelay12/1
  b(11)/1 -> BodyLSum11/1
  BodyLSum11/1 -> BodyLSum12/2
  BodyDelay12/1 -> b(12)/1, BodyDelay13/1
  b(12)/1 -> BodyLSum12/1
  BodyLSum12/1 -> BodyLSum13/2
  BodyDelay13/1 -> b(13)/1, BodyDelay14/1
  b(13)/1 -> BodyLSum13/1
  BodyLSum13/1 -> BodyLSum14/2
  BodyDelay14/1 -> b(14)/1, BodyDelay15/1
  b(14)/1 -> BodyLSum14/1
  BodyLSum14/1 -> BodyLSum15/2
  BodyDelay15/1 -> b(15)/1, BodyDelay16/1
  b(15)/1 -> BodyLSum15/1
  BodyLSum15/1 -> BodyLSum16/2
  BodyDelay16/1 -> b(16)/1, BodyDelay17/1
  b(16)/1 -> BodyLSum16/1
  BodyLSum16/1 -> BodyLSum17/2
  BodyDelay17/1 -> b(17)/1, BodyDelay18/1
  b(17)/1 -> BodyLSum17/1
  BodyLSum17/1 -> BodyLSum18/2
  BodyDelay18/1 -> b(18)/1, BodyDelay19/1
  b(18)/1 -> BodyLSum18/1
  BodyLSum18/1 -> BodyLSum19/2
  BodyDelay19/1 -> b(19)/1, BodyDelay20/1
  b(19)/1 -> BodyLSum19/1
  BodyLSum19/1 -> BodyLSum20/2
  BodyDelay20/1 -> b(20)/1, BodyDelay21/1
  b(20)/1 -> BodyLSum20/1
  BodyLSum20/1 -> BodyLSum21/2
  BodyDelay21/1 -> b(21)/1, BodyDelay22/1
  b(21)/1 -> BodyLSum21/1
  BodyLSum21/1 -> BodyLSum22/2
  BodyDelay22/1 -> b(22)/1, BodyDelay23/1
  b(22)/1 -> BodyLSum22/1
  BodyLSum22/1 -> BodyLSum23/2
  BodyDelay23/1 -> b(23)/1, BodyDelay24/1
  b(23)/1 -> BodyLSum23/1
  BodyLSum23/1 -> BodyLSum24/2
  BodyDelay24/1 -> b(24)/1, BodyDelay25/1
  b(24)/1 -> BodyLSum24/1
  BodyLSum24/1 -> BodyLSum25/2
  BodyDelay25/1 -> b(25)/1, BodyDelay26/1
  b(25)/1 -> BodyLSum25/1
  BodyLSum25/1 -> BodyLSum26/2
  BodyDelay26/1 -> b(26)/1, BodyDelay27/1
  b(26)/1 -> BodyLSum26/1
  BodyLSum26/1 -> BodyLSum27/2
  BodyDelay27/1 -> b(27)/1, BodyDelay28/1
  b(27)/1 -> BodyLSum27/1
  BodyLSum27/1 -> BodyLSum28/2
  BodyDelay28/1 -> b(28)/1, BodyDelay29/1
  b(28)/1 -> BodyLSum28/1
  BodyLSum28/1 -> BodyLSum29/2
  BodyDelay29/1 -> b(29)/1, BodyDelay30/1
  b(29)/1 -> BodyLSum29/1
  BodyLSum29/1 -> BodyLSum30/2
  BodyDelay30/1 -> b(30)/1, BodyDelay31/1
  b(30)/1 -> BodyLSum30/1
  BodyLSum30/1 -> BodyLSum31/2
  BodyDelay31/1 -> b(31)/1, BodyDelay32/1
  b(31)/1 -> BodyLSum31/1
  BodyLSum31/1 -> BodyLSum32/2
  BodyDelay32/1 -> b(32)/1, BodyDelay33/1
  b(32)/1 -> BodyLSum32/1
  BodyLSum32/1 -> BodyLSum33/2
  BodyDelay33/1 -> b(33)/1, BodyDelay34/1
  b(33)/1 -> BodyLSum33/1
  BodyLSum33/1 -> BodyLSum34/2
  BodyDelay34/1 -> b(34)/1, BodyDelay35/1
  b(34)/1 -> BodyLSum34/1
  BodyLSum34/1 -> BodyLSum35/2
  BodyDelay35/1 -> b(35)/1, BodyDelay36/1
  b(35)/1 -> BodyLSum35/1
  BodyLSum35/1 -> BodyLSum36/2
  BodyDelay36/1 -> b(36)/1, BodyDelay37/1
  b(36)/1 -> BodyLSum36/1
  BodyLSum36/1 -> BodyLSum37/2
  BodyDelay37/1 -> b(37)/1, BodyDelay38/1
  b(37)/1 -> BodyLSum37/1
  BodyLSum37/1 -> BodyLSum38/2
  BodyDelay38/1 -> b(38)/1, BodyDelay39/1
  b(38)/1 -> BodyLSum38/1
  BodyLSum38/1 -> BodyLSum39/2
  BodyDelay39/1 -> b(39)/1, BodyDelay40/1
  b(39)/1 -> BodyLSum39/1
  BodyLSum39/1 -> BodyLSum40/2
  BodyDelay40/1 -> b(40)/1, BodyDelay41/1
  b(40)/1 -> BodyLSum40/1
  BodyLSum40/1 -> BodyLSum41/2
  BodyDelay41/1 -> b(41)/1, BodyDelay42/1
  b(41)/1 -> BodyLSum41/1
  BodyLSum41/1 -> BodyLSum42/2
  BodyDelay42/1 -> b(42)/1, BodyDelay43/1
  b(42)/1 -> BodyLSum42/1
  BodyLSum42/1 -> BodyLSum43/2
  BodyDelay43/1 -> b(43)/1, BodyDelay44/1
  b(43)/1 -> BodyLSum43/1
  BodyLSum43/1 -> BodyLSum44/2
  BodyDelay44/1 -> b(44)/1, BodyDelay45/1
  b(44)/1 -> BodyLSum44/1
  BodyLSum44/1 -> BodyLSum45/2
  BodyDelay45/1 -> b(45)/1, BodyDelay46/1
  b(45)/1 -> BodyLSum45/1
  BodyLSum45/1 -> BodyLSum46/2
  BodyDelay46/1 -> b(46)/1, BodyDelay47/1
  b(46)/1 -> BodyLSum46/1
  BodyLSum46/1 -> BodyLSum47/2
  BodyDelay47/1 -> b(47)/1, BodyDelay48/1
  b(47)/1 -> BodyLSum47/1
  BodyLSum47/1 -> BodyLSum48/2
  BodyDelay48/1 -> b(48)/1, BodyDelay49/1
  b(48)/1 -> BodyLSum48/1
  BodyLSum48/1 -> BodyLSum49/2
  BodyDelay49/1 -> b(49)/1, BodyDelay50/1
  b(49)/1 -> BodyLSum49/1
  BodyLSum49/1 -> BodyLSum50/2
  BodyDelay50/1 -> b(50)/1, BodyDelay51/1
  b(50)/1 -> BodyLSum50/1
  BodyLSum50/1 -> BodyLSum51/2
  BodyDelay51/1 -> b(51)/1, BodyDelay52/1
  b(51)/1 -> BodyLSum51/1
  BodyLSum51/1 -> BodyLSum52/2
  BodyDelay52/1 -> b(52)/1, BodyDelay53/1
  b(52)/1 -> BodyLSum52/1
  BodyLSum52/1 -> BodyLSum53/2
  BodyDelay53/1 -> b(53)/1, BodyDelay54/1
  b(53)/1 -> BodyLSum53/1
  BodyLSum53/1 -> BodyLSum54/2
  BodyDelay54/1 -> b(54)/1, BodyDelay55/1
  b(54)/1 -> BodyLSum54/1
  BodyLSum54/1 -> BodyLSum55/1
  BodyDelay55/1 -> b(55)/1
  b(55)/1 -> BodyLSum55/2
  BodyLSum55/1 -> Output/1

== system Multi_Scenario_WECS_based_Microgrid_2017/Generator side control1/Discrete SV PWM Generator/SV Modulator Pattern #1/Generate pulse pattern/Determine interval of the PWM period based on Ta Tb and To ==
  TaTbTo : Inport
  Constant7 : Constant
  Demux1 : Demux  Outputs=6
      settings: DisplayOption=none
  Relational Operator{,1..5} (6 alike) : RelationalOperator  InputSameDT=off
  Subsystem : Subsystem
  Sum1 : Sum  Inputs=+++++++  SaturateOnIntegerOverflow=on
  Triangle : simulink/Sources/Repeating Sequence  rep_seq_t=[0 1/Fc]  rep_seq_y=[0 1/Fc]
  Tn : Outport
  wires:
  Sum1/1 -> Tn/1
  Demux1/6 -> Relational Operator4/2
  Demux1/5 -> Relational Operator3/2
  Demux1/4 -> Relational Operator2/2
  Demux1/3 -> Relational Operator1/2
  Demux1/2 -> Relational Operator/2
  Demux1/1 -> Relational Operator5/2
  Constant7/1 -> Sum1/1
  Relational Operator5/1 -> Sum1/2
  Relational Operator/1 -> Sum1/3
  Relational Operator1/1 -> Sum1/4
  Relational Operator2/1 -> Sum1/5
  Relational Operator3/1 -> Sum1/6
  Relational Operator4/1 -> Sum1/7
  Triangle/1 -> Relational Operator5/1, Relational Operator/1, Relational Operator1/1, Relational Operator2/1, Relational Operator3/1, Relational Operator4/1
  Subsystem/1(Timing) -> Demux1/1
  TaTbTo/1 -> Subsystem/1(TaTbTo)

== system Multi_Scenario_WECS_based_Microgrid_2017/Generator side control1/Discrete SV PWM Generator/SV Modulator Pattern #1/Generate pulse pattern/Determine interval of the PWM period based on Ta Tb and To/Subsystem ==
  TaTbTo : Inport
  "  1/2" : Gain  Gain=0.5  SaturateOnIntegerOverflow=on  OutDataTypeStr=Inherit: Same as input  ParamDataTypeStr=Inherit: Same as input
  " 1/2" : Gain  Gain=0.5  SaturateOnIntegerOverflow=on  OutDataTypeStr=Inherit: Same as input  ParamDataTypeStr=Inherit: Same as input
  " 1/2 " : Gain  Gain=0.5  SaturateOnIntegerOverflow=on  OutDataTypeStr=Inherit: Same as input  ParamDataTypeStr=Inherit: Same as input
  1/4 : Gain  Gain=0.25  SaturateOnIntegerOverflow=on  OutDataTypeStr=Inherit: Same as input  ParamDataTypeStr=Inherit: Same as input
  Demux : Demux  Outputs=3
      settings: DisplayOption=none
  Mux1 : Mux  Inputs=6
  Sum{5..9} (5 alike) : Sum  SaturateOnIntegerOverflow=on
  Timing : Outport
  wires:
  Mux1/1 -> Timing/1
  Sum5/1 -> Mux1/2, Sum6/1
  Sum6/1 -> Mux1/3, Sum7/1
  Sum7/1 -> Mux1/4, Sum8/1
  Sum8/1 -> Mux1/5, Sum9/1
  Sum9/1 -> Mux1/6
  1/4/1 -> Mux1/1, Sum5/1
  Demux/1 -> " 1/2 "/1
  Demux/2 -> "  1/2"/1
  " 1/2"/1 -> Sum7/2
  TaTbTo/1 -> Demux/1
  "  1/2"/1 -> Sum6/2, Sum8/2
  Demux/3 -> 1/4/1, " 1/2"/1
  " 1/2 "/1 -> Sum5/2, Sum9/2
